simulink model "monit_test2_cosim"  (Simulink 7.8)
settings: Solver=ode45  StartTime=0.0  StopTime=10e-4  RelTol=1e-3
undefined symbols (not defined in the file): A, frev_476, Fs_adc, N, n_ovs
libraries: simulink x2, xbsIndex_r4 x1, JTAGRuntimeCosim_r4 x1
settings Model: Creator=lucas.russo  LastModifiedBy=lucas.russo

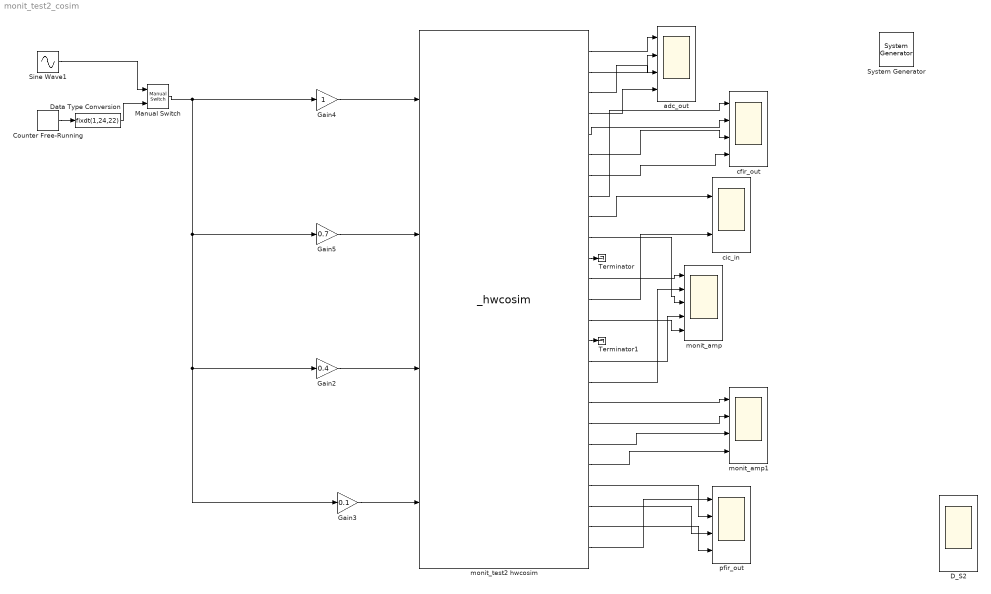
== system monit_test2_cosim ==
  " System Generator" : xbsIndex_r4/ System Generator  Tag=genX  xilinxfamily=virtex6  part=xc6vsx315t  speed=-3  package=ff1156  synthesis_tool=XST  clock_wrapper=Clock Enables  directory=./netlist  proj_type=Project Navigator  Synth_file=XST Defaults  Impl_file=ISE Defaults  testbench=off  simulink_period=1/Fs_adc/n_ovs  sysclk_period=1/Fs_adc/n_ovs*1e9  dcm_input_clock_period=10  incr_netlist=off  trim_vbits=Everywhere in SubSystem  dbl_ovrd=According to Block Masks  core_generation=According to Block Masks  run_coregen=off  deprecated_control=off  eval_field=0  block_type=sysgen
  Counter Free-Running : simulink/Sources/Counter Free-Running  NumBits=23  tsamp=-1
  D_S2 : Scope  NumInputPorts=5
      settings: TimeRange=0.0003  YMin=-1~2.76327e-005~-1~0.0622026~-5  YMax=1~3.05415e-005~1~0.0687502~5  SaveName=ScopeData6  MaxDataPoints=1000000  SampleInput=on
  Data Type Conversion : DataTypeConversion  OutDataTypeStr=fixdt(1,24,22)
  Gain2 : Gain  Gain=0.4
  Gain3 : Gain  Gain=0.1
  Gain4 : Gain
  Gain5 : Gain  Gain=0.7
  Manual Switch : simulink/Signal Routing/Manual Switch  sw=1  action=0  varsize=off
  Sine Wave1 : Sin  Frequency=2*pi*frev_476/476e6  SampleTime=0
  Terminator : Terminator
  Terminator1 : Terminator
  adc_out : Scope  NumInputPorts=4
      settings: TimeRange=0.0003  YMin=0.00018~0.000175~0.000125~0.000125  YMax=0.00029~0.0004~0.000375~0.00045  SaveName=ScopeData5  MaxDataPoints=1000000  SampleInput=on
  cfir_out : Scope  NumInputPorts=4
      settings: TimeRange=0.0003  YMin=-1~2.76327e-005~-1~0.0622026  YMax=1~3.05415e-005~1~0.0687502  SaveName=ScopeData2  MaxDataPoints=1000000  SampleInput=on
  cic_in : Scope  NumInputPorts=2
      settings: TimeRange=0.0003  YMin=-1~2.76327e-005  YMax=1~3.05415e-005  MaxDataPoints=1000000  SampleInput=on
  monit_amp : Scope  NumInputPorts=5
      settings: TimeRange=0.0002  YMin=-1~2.76327e-005~-1~0.0622026~-5  YMax=1~3.05415e-005~1~0.0687502~5  MaxDataPoints=1000000  SampleInput=on
  monit_amp1 : Scope  NumInputPorts=4
      settings: TimeRange=0.0003  YMin=-1~2.76327e-005~-1~0.0622026  YMax=1~3.05415e-005~1~0.0687502  SaveName=ScopeData3  MaxDataPoints=1000000  SampleInput=on
  monit_test2 hwcosim : JTAGRuntimeCosim_r4/_hwcosim  clkSrc=Single Stepped  hasCombinationalPath=on  bitfileName=D:\Sysgen_projects\ddc_bpm_476_066\models\tests\monit_test2_cosim\monit_test2_cw.bit  skipConfig=off  cable=Auto Detect  speed=N/A  cablePort=N/A  cableLocation=Local  shareCable=off  enable_codebug=on  design_xtable=|  engineDll=JTAGCosimEngine.dll  cableWaitTime=10  bscanPos=-1  IRLengths=[]  useWaitBox=1  hasBufgmux=on  Scheme=Cosim  useCmdProc=1  hasProc=0  block_type=jtagcosim
      | {
      |   'clkWrapper' => 'monit_test2_cw',
      |   'clocksGcd' => 1,
      |   'device' => 'xc6vlx240t-1ff1156',
      |   'ports' => {
      |     'adc_ch0_in' => {
      |       'bd_port_index' => 0,
      |       'direction' => 'in',
      |       'icon_text' => 'adc_ch0_in',
      |       'period' => 16,
      |       'proxy_name' => 'monit_test2/adc_ch0_in',
      |       'sim_pause_trigger' => false,
      |       'type' => 'Fix_24_22',
      |       'width' => 24,
      |     },
      |     'adc_ch0_out' => {
      |       'bd_port_index' => 0,
      |       'direction' => 'out',
      |       'icon_text' => 'adc_ch0_out',
      |       'period' => 16,
      |       'proxy_name' => 'monit_test2/adc_ch0_out',
      |       'sim_pause_trigger' => false,
      |       'type' => 'Fix_24_22',
      |       'width' => 24,
      |     },
      |     'adc_ch1_in' => {
      |       'bd_port_index' => 1,
      |       'direction' => 'in',
      |       'icon_text' => 'adc_ch1_in',
      |       'period' => 16,
      |       'proxy_name' => 'monit_test2/adc_ch1_in',
      |       'sim_pause_trigger' => false,
      |       'type' => 'Fix_24_22',
      |       'width' => 24,
      |     },
      |     'adc_ch1_out' => {
      |       'bd_port_index' => 1,
      |       'direction' => 'out',
      |       'icon_text' => 'adc_ch1_out',
      |       'period' => 16,
      |       'proxy_name' => 'monit_test2/adc_ch1_out',
      |       'sim_pause_trigger' => false,
      |       'type' => 'Fix_24_22',
      |       'width' => 24,
      |     },
      |     'adc_ch2_in' => {
      |       'bd_port_index' => 2,
      |       'direction' => 'in',
      |       'icon_text' => 'adc_ch2_in',
      |       'period' => 16,
      |       'proxy_name' => 'monit_test2/adc_ch2_in',
      |       'sim_pause_trigger' => false,
      |       'type' => 'Fix_24_22',
      |       'width' => 24,
      |     },
      |     'adc_ch2_out' => {
      |       'bd_port_index' => 2,
      |       'direction' => 'out',
      |       'icon_text' => 'adc_ch2_out',
      |       'period' => 16,
      |       'proxy_name' => 'monit_test2/adc_ch2_out',
      |       'sim_pause_trigger' => false,
      |       'type' => 'Fix_24_22',
      |       'width' => 24,
      |     },
      |     'adc_ch3_in' => {
      |       'bd_port_index' => 3,
      |       'direction' => 'in',
      |       'icon_text' => 'adc_ch3_in',
      |       'period' => 16,
      |       'proxy_name' => 'monit_test2/adc_ch3_in',
      |       'sim_pause_trigger' => false,
      |       'type' => 'Fix_24_22',
      |       'width' => 24,
      |     },
      |     'adc_ch3_out' => {
      |       'bd_port_index' => 3,
      |       'direction' => 'out',
      |       'icon_text' => 'adc_ch3_out',
      |       'period' => 16,
      |       'proxy_name' => 'monit_test2/adc_ch3_out',
      |       'sim_pause_trigger' => false,
      |       'type' => 'Fix_24_22',
      |       'width' => 24,
      |     },
      |     'cfir_chan_in_out' => {
      |       'bd_port_index' => 4,
      |       'direction' => 'out',
      |       'icon_text' => 'cfir_chan_in_out',
      |       'period' => 320,
      |       'proxy_name' => 'monit_test2/Monit_amp/Monit_amp_c/cfir_chan_in_out',
      |       'sim_pause_trigger' => false,
      |       'type' => 'UFix_2_0',
      |       'width' => 2,
      |     },
      |     'cfir_data_out' => {
      |       'bd_port_index' => 5,
      |       'direction' => 'out',
      |       'icon_text' => 'cfir_data_out',
      |       'period' => 320,
      |       'proxy_name' => 'monit_test2/Monit_amp/Monit_amp_c/cfir_data_out',
      |       'sim_pause_trigger' => false,
      |       'type' => 'Fix_25_21',
      |       'width' => 25,
      |     },
      |     'cfir_incorrect_out' => {
      |       'bd_port_index' => 6,
      |       'direction' => 'out',
      |       'icon_text' => 'cfir_incorrect_out',
      |       'period' => 160,
      |       'proxy_name' => 'monit_test2/Monit_amp/Monit_amp_c/cfir_incorrect_out',
      |       'sim_pause_trigger' => false,
      |       'type' => 'Bool',
      |       'width' => 1,
      |     },
      |     'cfir_valid_out' => {
      |       'bd_port_index' => 7,
      |       'direction' => 'out',
      |       'icon_text' => 'cfir_valid_out',
      |       'period' => 320,
      |       'proxy_name' => 'monit_test2/Monit_amp/Monit_amp_c/cfir_valid_out',
      |       'sim_pause_trigger' => false,
      |       'type' => 'Bool',
      |       'width' => 1,
      |     },
      |     'cic_ch_in' => {
      |       'bd_port_index' => 8,
      |       'direction' => 'out',
      |       'icon_text' => 'cic_ch_in',
      |       'period' => 4,
      |       'proxy_name' => 'monit_test2/Monit_amp/Monit_amp_c/cic_ch_in',
      |       'sim_pause_trigger' => false,
      |       'type' => 'UFix_2_0',
      |       'width' => 2,
      |     },
      |     'cic_ch_out' => {
      |       'bd_port_index' => 9,
      |       'direction' => 'out',
      |       'icon_text' => 'cic_ch_out',
      |       'period' => 160,
      |       'proxy_name' => 'monit_test2/Monit_amp/Monit_amp_c/cic_ch_out',
      |       'sim_pause_trigger' => false,
      |       'type' => 'UFix_2_0',
      |       'width' => 2,
      |     },
      |     'cic_chan_sync_out' => {
      |       'bd_port_index' => 10,
      |       'direction' => 'out',
      |       'icon_text' => 'cic_chan_sync_out',
      |       'period' => 160,
      |       'proxy_name' => 'monit_test2/Monit_amp/Monit_amp_c/cic_chan_sync_out',
      |       'sim_pause_trigger' => false,
      |       'type' => 'UFix_1_0',
      |       'width' => 1,
      |     },
      |     'cic_data_out' => {
      |       'bd_port_index' => 11,
      |       'direction' => 'out',
      |       'icon_text' => 'cic_data_out',
      |       'period' => 160,
      |       'proxy_name' => 'monit_test2/Monit_amp/Monit_amp_c/cic_data_out',
      |       'sim_pause_trigger' => false,
      |       'type' => 'Fix_25_0',
      |       'width' => 25,
      |     },
      |     'cic_last' => {
      |       'bd_port_index' => 12,
      |       'direction' => 'out',
      |       'icon_text' => 'cic_last',
      |       'period' => 4,
      |       'proxy_name' => 'monit_test2/Monit_amp/Monit_amp_c/cic_last',
      |       'sim_pause_trigger' => false,
      |       'type' => 'Bool',
      |       'width' => 1,
      |     },
      |     'cic_last_missing_out' => {
      |       'bd_port_index' => 13,
      |       'direction' => 'out',
      |       'icon_text' => 'cic_last_missing_out',
      |       'period' => 4,
      |       'proxy_name' => 'monit_test2/Monit_amp/Monit_amp_c/cic_last_missing_out',
      |       'sim_pause_trigger' => false,
      |       'type' => 'Bool',
      |       'width' => 1,
      |     },
      |     'cic_last_out' => {
      |       'bd_port_index' => 14,
      |       'direction' => 'out',
      |       'icon_text' => 'cic_last_out',
      |       'period' => 160,
      |       'proxy_name' => 'monit_test2/Monit_amp/Monit_amp_c/cic_last_out',
      |       'sim_pause_trigger' => false,
      |       'type' => 'Bool',
      |       'width' => 1,
      |     },
      |     'cic_unexpected' => {
      |       'bd_port_index' => 15,
      |       'direction' => 'out',
      |       'icon_text' => 'cic_unexpected',
      |       'period' => 4,
      |       'proxy_name' => 'monit_test2/Monit_amp/Monit_amp_c/cic_unexpected',
      |       'sim_pause_trigger' => false,
      |       'type' => 'Bool',
      |       'width' => 1,
      |     },
      |     'cic_valid_out' => {
      |       'bd_port_index' => 16,
      |       'direction' => 'out',
      |       'icon_text' => 'cic_valid_out',
      |       'period' => 160,
      |       'proxy_name' => 'monit_test2/Monit_amp/Monit_amp_c/cic_valid_out',
      |       'sim_pause_trigger' => false,
      |       'type' => 'Bool',
      |       'width' => 1,
      |     },
      |     'monit_amp_ch0_out' => {
      |       'bd_port_index' => 17,
      |       'direction' => 'out',
      |       'icon_text' => 'monit_amp_ch0_out',
      |       'period' => 2560,
      |       'proxy_name' => 'monit_test2/monit_amp_ch0_out',
      |       'sim_pause_trigger' => false,
      |       'type' => 'Fix_24_22',
      |       'width' => 24,
      |     },
      |     'monit_amp_ch1_out' => {
      |       'bd_port_index' => 18,
      |       'direction' => 'out',
      |       'icon_text' => 'monit_amp_ch1_out',
      |       'period' => 2560,
      |       'proxy_name' => 'monit_test2/monit_amp_ch1_out',
      |       'sim_pause_trigger' => false,
      |       'type' => 'Fix_24_22',
      |       'width' => 24,
      |     },
      |     'monit_amp_ch2_out' => {
      |       'bd_port_index' => 19,
      |       'direction' => 'out',
      |       'icon_text' => 'monit_amp_ch2_out',
      |       'period' => 2560,
      |       'proxy_name' => 'monit_test2/monit_amp_ch2_out',
      |       'sim_pause_trigger' => false,
      |       'type' => 'Fix_24_22',
      |       'width' => 24,
      |     },
      |     'monit_amp_ch3_out' => {
      |       'bd_port_index' => 20,
      |       'direction' => 'out',
      |       'icon_text' => 'monit_amp_ch3_out',
      |       'period' => 2560,
      |       'proxy_name' => 'monit_test2/monit_amp_ch3_out',
      |       'sim_pause_trigger' => false,
      |       'type' => 'Fix_24_22',
      |       'width' => 24,
      |     },
      |     'pfir_chain_id_out' => {
      |       'bd_port_index' => 21,
      |       'direction' => 'out',
      |       'icon_text' => 'pfir_chain_id_out',
      |       'period' => 640,
      |       'proxy_name' => 'monit_test2/Monit_amp/Monit_amp_c/pfir_chain_id_out',
      |       'sim_pause_trigger' => false,
      |       'type' => 'UFix_2_0',
      |       'width' => 2,
      |     },
      |     'pfir_data_out' => {
      |       'bd_port_index' => 22,
      |       'direction' => 'out',
      |       'icon_text' => 'pfir_data_out',
      |       'period' => 640,
      |       'proxy_name' => 'monit_test2/Monit_amp/Monit_amp_c/pfir_data_out',
      |       'sim_pause_trigger' => false,
      |       'type' => 'Fix_25_21',
      |       'width' => 25,
      |     },
      |     'pfir_incorrect_out' => {
      |       'bd_port_index' => 23,
      |       'direction' => 'out',
      |       'icon_text' => 'pfir_incorrect_out',
      |       'period' => 320,
      |       'proxy_name' => 'monit_test2/Monit_amp/Monit_amp_c/pfir_incorrect_out',
      |       'sim_pause_trigger' => false,
      |       'type' => 'Bool',
      |       'width' => 1,
      |     },
      |     'pfir_valid_out' => {
      |       'bd_port_index' => 24,
      |       'direction' => 'out',
      |       'icon_text' => 'pfir_valid_out',
      |       'period' => 640,
      |       'proxy_name' => 'monit_test2/Monit_amp/Monit_amp_c/pfir_valid_out',
      |       'sim_pause_trigger' => false,
      |       'type' => 'Bool',
      |       'width' => 1,
      |     },
      |   },
      |   'shared_memories' => {},
      | }
  pfir_out : Scope  NumInputPorts=4
      settings: TimeRange=0.0003  YMin=-1~2.76327e-005~-1~0.0622026  YMax=1~3.05415e-005~1~0.0687502  SaveName=ScopeData4  MaxDataPoints=1000000  SampleInput=on
  wires:
  monit_test2 hwcosim/1 -> adc_out/1
  monit_test2 hwcosim/2 -> adc_out/2
  monit_test2 hwcosim/3 -> adc_out/3
  monit_test2 hwcosim/4 -> adc_out/4
  monit_test2 hwcosim/9 -> cic_in/1
  monit_test2 hwcosim/13 -> cic_in/2
  monit_test2 hwcosim/12 -> monit_amp/1
  monit_test2 hwcosim/17 -> monit_amp/2
  monit_test2 hwcosim/10 -> monit_amp/3
  monit_test2 hwcosim/16 -> monit_amp/4
  monit_test2 hwcosim/14 -> monit_amp/5
  monit_test2 hwcosim/8 -> cfir_out/1
  monit_test2 hwcosim/5 -> cfir_out/2
  monit_test2 hwcosim/6 -> cfir_out/3
  monit_test2 hwcosim/7 -> cfir_out/4
  monit_test2 hwcosim/18 -> monit_amp1/1
  monit_test2 hwcosim/19 -> monit_amp1/2
  monit_test2 hwcosim/20 -> monit_amp1/3
  monit_test2 hwcosim/21 -> monit_amp1/4
  monit_test2 hwcosim/25 -> pfir_out/1
  monit_test2 hwcosim/22 -> pfir_out/2
  monit_test2 hwcosim/23 -> pfir_out/3
  monit_test2 hwcosim/24 -> pfir_out/4
  Sine Wave1/1 -> Manual Switch/1
  Counter Free-Running/1 -> Data Type Conversion/1
  Manual Switch/1 -> Gain4/1, Gain2/1, Gain3/1, Gain5/1
  Data Type Conversion/1 -> Manual Switch/2
  Gain3/1 -> monit_test2 hwcosim/4
  Gain2/1 -> monit_test2 hwcosim/3
  Gain5/1 -> monit_test2 hwcosim/2
  Gain4/1 -> monit_test2 hwcosim/1
  monit_test2 hwcosim/11 -> Terminator/1
  monit_test2 hwcosim/15 -> Terminator1/1
